simulink model "SWC_ADM"  (R2020a)
settings: Solver=FixedStepDiscrete  StartTime=0.0  StopTime=10  FixedStep=0.001  RelTol=1e-3
values from neighbouring files (symbols this model uses):
  CAL_ADM_BMSLowerThr_f32 = 0.0    [SWC_ADM_DataDictionary.sldd]
  CAL_ADM_BMSUpperThr_f32 = 0.0    [SWC_ADM_DataDictionary.sldd]
  CAL_ADM_BMSVoltRngErrCntThr_s16 = 0.0    [SWC_ADM_DataDictionary.sldd]
  CAL_ADM_BMSVoltRngErrDebThr_s16 = 0.0    [SWC_ADM_DataDictionary.sldd]
  CAL_ADM_BMSVoltRngErrRst_b = 0.0    [SWC_ADM_DataDictionary.sldd]
  CAL_ADM_DchgMode_u8 = 0.0    [SWC_ADM_DataDictionary.sldd]
  CAL_ADM_flgCrash_b = 0.0    [SWC_ADM_DataDictionary.sldd]
  CAL_ADM_flgCrashSwt_b = 0.0    [SWC_ADM_DataDictionary.sldd]
  CAL_ADM_flgDchgReq_b = 0.0    [SWC_ADM_DataDictionary.sldd]
  CAL_ADM_flgDchgReqSwt_b = 0.0    [SWC_ADM_DataDictionary.sldd]
  CAL_ADM_flgstModeReqSwt_b = 0.0    [SWC_ADM_DataDictionary.sldd]
  CAL_ADM_GlbDchgErrRst_b = 0.0    [SWC_ADM_DataDictionary.sldd]
  CAL_ADM_GlbDchgThrshTime_f32 = 0.0    [SWC_ADM_DataDictionary.sldd]
  CAL_ADM_GlbDchgThrshVolt_f32 = 0.0    [SWC_ADM_DataDictionary.sldd]
  CAL_ADM_L2Com_BMSVolt = 0.0    [SWC_ADM_DataDictionary.sldd]
  CAL_ADM_L2Com_BMSVolt_b = 0.0    [SWC_ADM_DataDictionary.sldd]
  CAL_ADM_L2Com_HiPrecVolt = 0.0    [SWC_ADM_DataDictionary.sldd]
  CAL_ADM_L2Com_HiPrecVolt_b = 0.0    [SWC_ADM_DataDictionary.sldd]
  CAL_ADM_stModeReq_u8 = 0.0    [SWC_ADM_DataDictionary.sldd]
  CAL_ADM_VoltAbsDiffThr_f32 = 0.0    [SWC_ADM_DataDictionary.sldd]
  CAL_ADM_VoltAbsDiffThrPerc_f32 = 0.0    [SWC_ADM_DataDictionary.sldd]
  CAL_ADM_VoltChgThr_f32 = 0.0    [SWC_ADM_DataDictionary.sldd]
  CAL_ADM_VoltCmpChkErrCntThr_s16 = 0.0    [SWC_ADM_DataDictionary.sldd]
  CAL_ADM_VoltCmpChkErrDebThr_s16 = 0.0    [SWC_ADM_DataDictionary.sldd]
  CAL_ADM_VoltCmpChkErrRst_b = 0.0    [SWC_ADM_DataDictionary.sldd]
  CAL_ADM_VoltCmpChkErrst_b = 0.0    [SWC_ADM_DataDictionary.sldd]
libraries: simulink x2
settings Model: DataDictionary=SWC_ADM_DataDictionary.sldd  Creator=wangzeda  LastModifiedBy=yangxinqiao
settings DataIOCC: SaveFormat=StructureWithTime
settings OptimizationCC: DefaultParameterBehavior=Inlined  DefaultUnderspecifiedDataType=single  EnhancedBackFolding=on  PassReuseOutputArgsAs=Individual arguments  ZeroExternalMemoryAtStartup=off  ZeroInternalMemoryAtStartup=off  OptimizeBlockOrder=speed  DifferentSizesBufferReuse=on  OptimizationCustomize=off  EfficientTunableParamExpr=on
settings DebuggingCC: ParameterTunabilityLossMsg=error
settings ModelReferenceCC: ModelReferenceNumInstancesAllowed=Single
settings SFSimCC: MATLABDynamicMemAlloc=off
settings RTWCC: SystemTargetFile=ert.tlc  GenCodeOnly=on  TemplateMakefile=ert_default_tmf  CustomSourceCode="#include \"set_get_data.h\""
settings CodeAppCC: ForceParamTrailComments=on  IgnoreCustomStorageClasses=off  OperatorAnnotations=on  SimulinkDataObjDesc=on  SFDataObjDesc=on  InsertBlockDesc=on
settings ERTTargetCC: TargetLangStandard=C99 (ISO)  GenerateASAP2=on  InlinedParameterPlacement=NonHierarchical  ERTCustomFileTemplate=example_file_process.tlc  EnableUserReplacementTypes=on

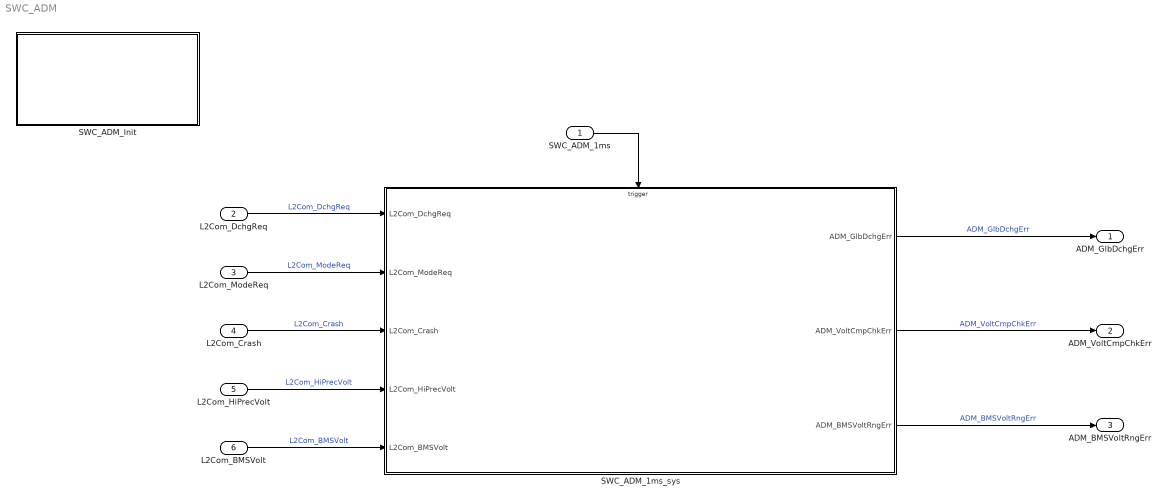
== system SWC_ADM ==
  SWC_ADM_1ms : Inport  SampleTime=0.001  OutputFunctionCall=on
  L2Com_DchgReq : Inport  Port=2  OutDataTypeStr=boolean  PortDimensions=1
  L2Com_ModeReq : Inport  Port=3  OutDataTypeStr=uint8  PortDimensions=1
  L2Com_Crash : Inport  Port=4  OutDataTypeStr=boolean  PortDimensions=1
  L2Com_HiPrecVolt : Inport  Port=5  OutDataTypeStr=single  PortDimensions=1
  L2Com_BMSVolt : Inport  Port=6  OutDataTypeStr=single  PortDimensions=1
  SWC_ADM_1ms_sys : Subsystem
  SWC_ADM_Init : Subsystem
  ADM_GlbDchgErr : Outport  OutDataTypeStr=boolean  PortDimensions=1
  ADM_VoltCmpChkErr : Outport  Port=2  OutDataTypeStr=boolean  OutputWhenDisabled=reset  InitialOutput=[0]  VectorParamsAs1DForOutWhenUnconnected=off
  ADM_BMSVoltRngErr : Outport  Port=3  OutDataTypeStr=boolean  PortDimensions=1
  wires:
  L2Com_Crash/1 -> SWC_ADM_1ms_sys/3(L2Com_Crash)  "L2Com_Crash"
  L2Com_BMSVolt/1 -> SWC_ADM_1ms_sys/5(L2Com_BMSVolt)  "L2Com_BMSVolt"
  SWC_ADM_1ms_sys/1(ADM_GlbDchgErr) -> ADM_GlbDchgErr/1  "ADM_GlbDchgErr"
  SWC_ADM_1ms/1 -> SWC_ADM_1ms_sys/Trigger
  L2Com_ModeReq/1 -> SWC_ADM_1ms_sys/2(L2Com_ModeReq)  "L2Com_ModeReq"
  L2Com_DchgReq/1 -> SWC_ADM_1ms_sys/1(L2Com_DchgReq)  "L2Com_DchgReq"
  SWC_ADM_1ms_sys/3(ADM_BMSVoltRngErr) -> ADM_BMSVoltRngErr/1  "ADM_BMSVoltRngErr"
  L2Com_HiPrecVolt/1 -> SWC_ADM_1ms_sys/4(L2Com_HiPrecVolt)  "L2Com_HiPrecVolt"
  SWC_ADM_1ms_sys/2(ADM_VoltCmpChkErr) -> ADM_VoltCmpChkErr/1  "ADM_VoltCmpChkErr"

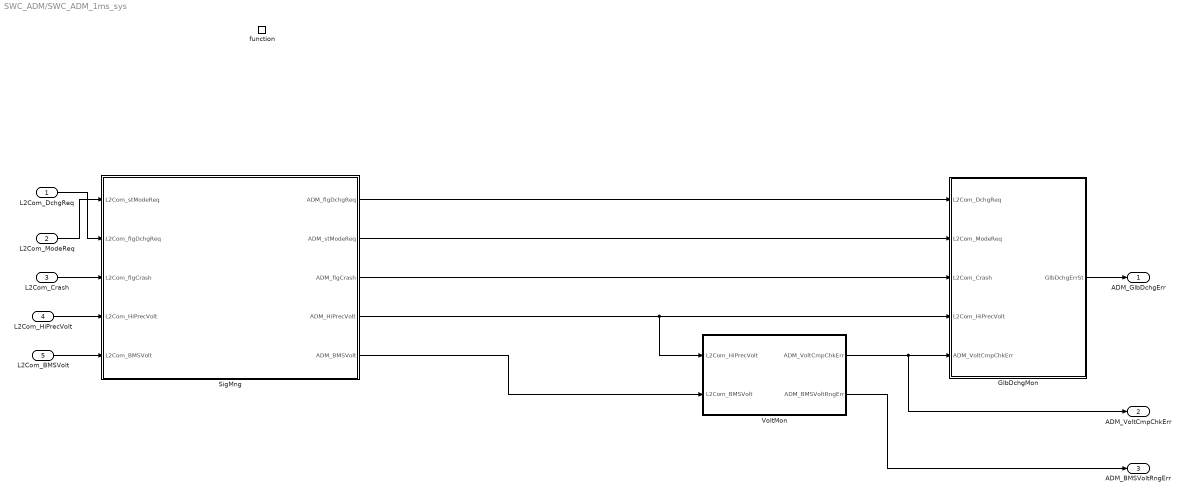
== system SWC_ADM/SWC_ADM_1ms_sys ==
  L2Com_DchgReq : Inport
  L2Com_ModeReq : Inport  Port=2
  L2Com_Crash : Inport  Port=3
  L2Com_HiPrecVolt : Inport  Port=4
  L2Com_BMSVolt : Inport  Port=5
  function : TriggerPort  TriggerType=function-call  VariantControl=(inherit)  SampleTimeType=periodic  SampleTime=-1
  GlbDchgMon : Subsystem  TreatAsAtomicUnit=on
      settings: RTWSystemCode=Nonreusable function
  SigMng : Subsystem  TreatAsAtomicUnit=on
  VoltMon : Subsystem
      settings: RTWSystemCode=Nonreusable function
  ADM_GlbDchgErr : Outport  VectorParamsAs1DForOutWhenUnconnected=off
  ADM_VoltCmpChkErr : Outport  Port=2  OutDataTypeStr=boolean  OutputWhenDisabled=reset  InitialOutput=[0]  VectorParamsAs1DForOutWhenUnconnected=off
  ADM_BMSVoltRngErr : Outport  Port=3  VectorParamsAs1DForOutWhenUnconnected=off
  wires:
  GlbDchgMon/1(GlbDchgErrSt) -> ADM_GlbDchgErr/1
  VoltMon/2(ADM_BMSVoltRngErr) -> ADM_BMSVoltRngErr/1
  VoltMon/1(ADM_VoltCmpChkErr) -> ADM_VoltCmpChkErr/1, GlbDchgMon/5(ADM_VoltCmpChkErr)
  SigMng/3(ADM_flgCrash) -> GlbDchgMon/3(L2Com_Crash)
  SigMng/2(ADM_stModeReq) -> GlbDchgMon/2(L2Com_ModeReq)
  SigMng/1(ADM_flgDchgReq) -> GlbDchgMon/1(L2Com_DchgReq)
  SigMng/4(ADM_HiPrecVolt) -> VoltMon/1(L2Com_HiPrecVolt), GlbDchgMon/4(L2Com_HiPrecVolt)
  SigMng/5(ADM_BMSVolt) -> VoltMon/2(L2Com_BMSVolt)
  L2Com_DchgReq/1 -> SigMng/2(L2Com_flgDchgReq)
  L2Com_ModeReq/1 -> SigMng/1(L2Com_stModeReq)
  L2Com_Crash/1 -> SigMng/3(L2Com_flgCrash)
  L2Com_HiPrecVolt/1 -> SigMng/4(L2Com_HiPrecVolt)
  L2Com_BMSVolt/1 -> SigMng/5(L2Com_BMSVolt)

== system SWC_ADM/SWC_ADM_Init ==
  Event Listener : EventListener  EventName=reset

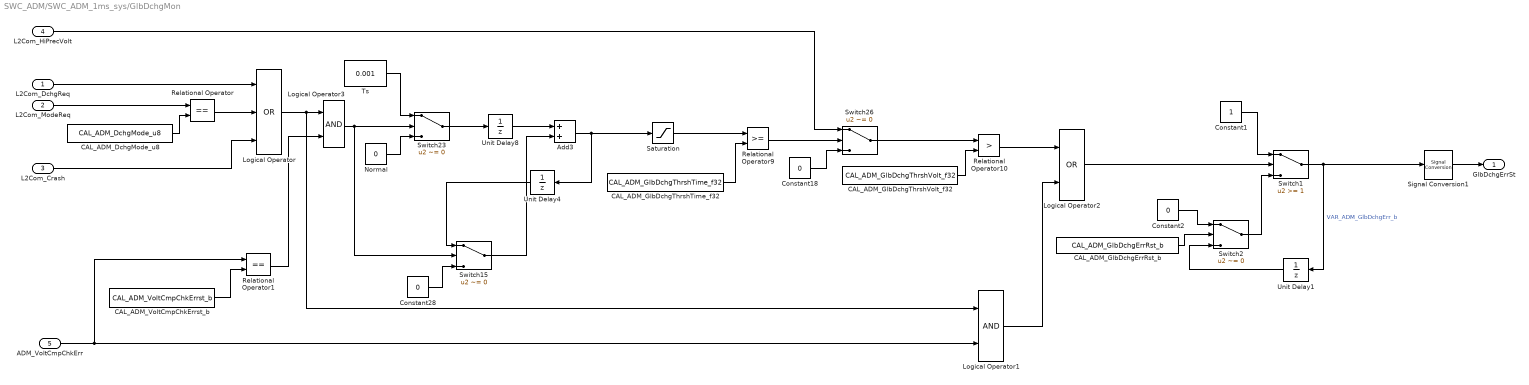
== system SWC_ADM/SWC_ADM_1ms_sys/GlbDchgMon ==
  L2Com_DchgReq : Inport
  L2Com_ModeReq : Inport  Port=2
  L2Com_Crash : Inport  Port=3
  L2Com_HiPrecVolt : Inport  Port=4
  ADM_VoltCmpChkErr : Inport  Port=5
  Add3 : Sum  AccumDataTypeStr=single
  CAL_ADM_DchgMode_u8 : Constant  Value=CAL_ADM_DchgMode_u8
  CAL_ADM_GlbDchgErrRst_b : Constant  Value=CAL_ADM_GlbDchgErrRst_b
  CAL_ADM_GlbDchgThrshTime_f32 : Constant  Value=CAL_ADM_GlbDchgThrshTime_f32
  CAL_ADM_GlbDchgThrshVolt_f32 : Constant  Value=CAL_ADM_GlbDchgThrshVolt_f32
  CAL_ADM_VoltCmpChkErrst_b : Constant  Value=CAL_ADM_VoltCmpChkErrst_b
  Constant1 : Constant  OutDataTypeStr=boolean
  Constant18 : Constant  Value=0
  Constant2 : Constant  Value=0  OutDataTypeStr=boolean
  Constant28 : Constant  Value=0
  Logical Operator : Logic  Operator=OR  Inputs=3  AllPortsSameDT=off  OutDataTypeStr=boolean
  Logical Operator1 : Logic  AllPortsSameDT=off  OutDataTypeStr=boolean
  Logical Operator2 : Logic  Operator=OR  AllPortsSameDT=off  OutDataTypeStr=boolean
  Logical Operator3 : Logic  AllPortsSameDT=off  OutDataTypeStr=boolean
  Normal : Constant  Value=0
  Relational Operator : RelationalOperator  Operator===  OutDataTypeStr=boolean  RndMeth=Simplest
  Relational Operator1 : RelationalOperator  Operator===  OutDataTypeStr=boolean  RndMeth=Simplest
  Relational Operator10 : RelationalOperator  Operator=>  OutDataTypeStr=boolean  RndMeth=Simplest
  Relational Operator9 : RelationalOperator  OutDataTypeStr=boolean  RndMeth=Simplest
  Saturation : Saturate  UpperLimit=3  LowerLimit=0
  Signal Conversion1 : SignalConversion  OverrideOpt=off
  Switch1 : Switch  Threshold=1
  Switch15 : Switch  Criteria=u2 ~= 0  OutDataTypeStr=single
  Switch2 : Switch  Criteria=u2 ~= 0
  Switch23 : Switch  Criteria=u2 ~= 0  OutDataTypeStr=single
  Switch26 : Switch  Criteria=u2 ~= 0  OutDataTypeStr=single
  Ts : Constant  Value=0.001
  Unit Delay1 : UnitDelay  SampleTime=-1  HasFrameUpgradeWarning=on
  Unit Delay4 : UnitDelay  SampleTime=-1  HasFrameUpgradeWarning=on
  Unit Delay8 : UnitDelay  SampleTime=-1  HasFrameUpgradeWarning=on
  GlbDchgErrSt : Outport  OutDataTypeStr=boolean  OutputWhenDisabled=reset  InitialOutput=[0]  VectorParamsAs1DForOutWhenUnconnected=off
  wires:
  Switch26/1 -> Relational Operator10/1
  Unit Delay4/1 -> Switch15/1
  Constant18/1 -> Switch26/3
  CAL_ADM_GlbDchgThrshVolt_f32/1 -> Relational Operator10/2
  Unit Delay8/1 -> Add3/1
  Logical Operator/1 -> Logical Operator1/1, Logical Operator3/1
  Constant28/1 -> Switch15/3
  Unit Delay1/1 -> Switch2/3
  Add3/1 -> Saturation/1, Unit Delay4/1
  Switch15/1 -> Add3/2
  Switch23/1 -> Unit Delay8/1
  Normal/1 -> Switch23/3
  Ts/1 -> Switch23/1
  Saturation/1 -> Relational Operator9/1
  CAL_ADM_GlbDchgThrshTime_f32/1 -> Relational Operator9/2
  Constant2/1 -> Switch2/1
  CAL_ADM_GlbDchgErrRst_b/1 -> Switch2/2
  L2Com_HiPrecVolt/1 -> Switch26/1
  Relational Operator10/1 -> Logical Operator2/1
  Signal Conversion1/1 -> GlbDchgErrSt/1
  Relational Operator9/1 -> Switch26/2
  L2Com_DchgReq/1 -> Logical Operator/1
  CAL_ADM_DchgMode_u8/1 -> Relational Operator/2
  L2Com_Crash/1 -> Logical Operator/3
  Relational Operator/1 -> Logical Operator/2
  L2Com_ModeReq/1 -> Relational Operator/1
  ADM_VoltCmpChkErr/1 -> Logical Operator1/2, Relational Operator1/1
  Logical Operator1/1 -> Logical Operator2/2
  Switch1/1 -> Unit Delay1/1, Signal Conversion1/1  "VAR_ADM_GlbDchgErr_b"
  CAL_ADM_VoltCmpChkErrst_b/1 -> Relational Operator1/2
  Relational Operator1/1 -> Logical Operator3/2
  Logical Operator3/1 -> Switch15/2, Switch23/2
  Logical Operator2/1 -> Switch1/2
  Constant1/1 -> Switch1/1
  Switch2/1 -> Switch1/3

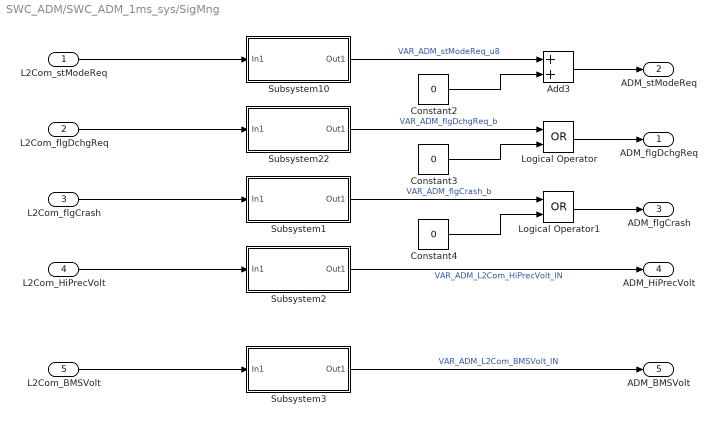
== system SWC_ADM/SWC_ADM_1ms_sys/SigMng ==
  L2Com_stModeReq : Inport
  L2Com_flgDchgReq : Inport  Port=2
  L2Com_flgCrash : Inport  Port=3
  L2Com_HiPrecVolt : Inport  Port=4
  L2Com_BMSVolt : Inport  Port=5
  Add3 : Sum
  Constant2 : Constant  Value=0  OutDataTypeStr=uint8
  Constant3 : Constant  Value=0  OutDataTypeStr=boolean
  Constant4 : Constant  Value=0  OutDataTypeStr=boolean
  Logical Operator : Logic  Operator=OR  AllPortsSameDT=off  OutDataTypeStr=boolean
  Logical Operator1 : Logic  Operator=OR  AllPortsSameDT=off  OutDataTypeStr=boolean
  Subsystem1 : Subsystem  mask{Switch_C=CAL_ADM_flgCrashSwt_b, Phy_Signal_C=CAL_ADM_flgCrash_b}
      mask prompts: Switch_C "Swich_C"
  Subsystem10 : Subsystem  mask{Switch_C=CAL_ADM_flgstModeReqSwt_b, Phy_Signal_C=CAL_ADM_stModeReq_u8}
      mask prompts: Switch_C "Swich_C"
  Subsystem2 : Subsystem  mask{Switch_C=CAL_ADM_L2Com_HiPrecVolt_b, Phy_Signal_C=CAL_ADM_L2Com_HiPrecVolt}
      mask prompts: Switch_C "Swich_C"
  Subsystem22 : Subsystem  mask{Switch_C=CAL_ADM_flgDchgReqSwt_b, Phy_Signal_C=CAL_ADM_flgDchgReq_b}
      mask prompts: Switch_C "Swich_C"
  Subsystem3 : Subsystem  mask{Switch_C=CAL_ADM_L2Com_BMSVolt_b, Phy_Signal_C=CAL_ADM_L2Com_BMSVolt}
      mask prompts: Switch_C "Swich_C"
  ADM_flgDchgReq : Outport  OutDataTypeStr=boolean  PortDimensions=1
  ADM_stModeReq : Outport  Port=2  OutDataTypeStr=uint8  PortDimensions=1
  ADM_flgCrash : Outport  Port=3  OutDataTypeStr=boolean  PortDimensions=1
  ADM_HiPrecVolt : Outport  Port=4
  ADM_BMSVolt : Outport  Port=5
  wires:
  Subsystem1/1(Out1) -> Logical Operator1/1  "VAR_ADM_flgCrash_b"
  Add3/1 -> ADM_stModeReq/1
  L2Com_flgCrash/1 -> Subsystem1/1(In1)
  Constant3/1 -> Logical Operator/2
  L2Com_flgDchgReq/1 -> Subsystem22/1(In1)
  Constant2/1 -> Add3/2
  Logical Operator/1 -> ADM_flgDchgReq/1
  Constant4/1 -> Logical Operator1/2
  Logical Operator1/1 -> ADM_flgCrash/1
  L2Com_stModeReq/1 -> Subsystem10/1(In1)
  Subsystem10/1(Out1) -> Add3/1  "VAR_ADM_stModeReq_u8"
  Subsystem22/1(Out1) -> Logical Operator/1  "VAR_ADM_flgDchgReq_b"
  L2Com_HiPrecVolt/1 -> Subsystem2/1(In1)
  Subsystem2/1(Out1) -> ADM_HiPrecVolt/1  "VAR_ADM_L2Com_HiPrecVolt_IN"
  L2Com_BMSVolt/1 -> Subsystem3/1(In1)
  Subsystem3/1(Out1) -> ADM_BMSVolt/1  "VAR_ADM_L2Com_BMSVolt_IN"

== system SWC_ADM/SWC_ADM_1ms_sys/VoltMon ==
  L2Com_HiPrecVolt : Inport
  L2Com_BMSVolt : Inport  Port=2
  BMSVoltRngMon : Subsystem
      settings: RTWSystemCode=Nonreusable function
  VoltCmpChkMon : Subsystem
      settings: RTWSystemCode=Nonreusable function
  ADM_VoltCmpChkErr : Outport  OutDataTypeStr=boolean  OutputWhenDisabled=reset  InitialOutput=[0]  VectorParamsAs1DForOutWhenUnconnected=off
  ADM_BMSVoltRngErr : Outport  Port=2  OutDataTypeStr=boolean  OutputWhenDisabled=reset  InitialOutput=[0]  VectorParamsAs1DForOutWhenUnconnected=off
  wires:
  BMSVoltRngMon/1(ADM_BMSVoltRngErr) -> ADM_BMSVoltRngErr/1
  L2Com_HiPrecVolt/1 -> VoltCmpChkMon/1(L2Com_HiPrecVolt)
  VoltCmpChkMon/1(ADM_VoltCmpChkErr) -> ADM_VoltCmpChkErr/1
  L2Com_BMSVolt/1 -> BMSVoltRngMon/1(L2Com_BMSVolt), VoltCmpChkMon/2(L2Com_BMSVolt)

== system SWC_ADM/SWC_ADM_1ms_sys/SigMng/Subsystem1 ==
  In1 : Inport
  Constant2 : Constant  Value=Switch_C  OutDataTypeStr=boolean
  Constant3 : Constant  Value=Phy_Signal_C
  Data Type Conversion : DataTypeConversion
  Switch : Switch  Criteria=u2 ~= 0
  Out1 : Outport  VectorParamsAs1DForOutWhenUnconnected=off
  wires:
  Data Type Conversion/1 -> Switch/3
  Constant3/1 -> Switch/1
  In1/1 -> Data Type Conversion/1
  Constant2/1 -> Switch/2
  Switch/1 -> Out1/1

== system SWC_ADM/SWC_ADM_1ms_sys/SigMng/Subsystem10 ==
  In1 : Inport
  Constant2 : Constant  Value=Switch_C  OutDataTypeStr=boolean
  Constant3 : Constant  Value=Phy_Signal_C
  Data Type Conversion : DataTypeConversion
  Switch : Switch  Criteria=u2 ~= 0
  Out1 : Outport  VectorParamsAs1DForOutWhenUnconnected=off
  wires:
  Switch/1 -> Out1/1
  Constant2/1 -> Switch/2
  In1/1 -> Data Type Conversion/1
  Constant3/1 -> Switch/1
  Data Type Conversion/1 -> Switch/3

== system SWC_ADM/SWC_ADM_1ms_sys/SigMng/Subsystem2 ==
  In1 : Inport
  Constant2 : Constant  Value=Switch_C  OutDataTypeStr=boolean
  Constant3 : Constant  Value=Phy_Signal_C
  Data Type Conversion : DataTypeConversion
  Switch : Switch  Criteria=u2 ~= 0
  Out1 : Outport  VectorParamsAs1DForOutWhenUnconnected=off
  wires:
  Data Type Conversion/1 -> Switch/3
  Constant3/1 -> Switch/1
  In1/1 -> Data Type Conversion/1
  Constant2/1 -> Switch/2
  Switch/1 -> Out1/1

== system SWC_ADM/SWC_ADM_1ms_sys/SigMng/Subsystem22 ==
  In1 : Inport
  Constant2 : Constant  Value=Switch_C  OutDataTypeStr=boolean
  Constant3 : Constant  Value=Phy_Signal_C
  Data Type Conversion : DataTypeConversion
  Switch : Switch  Criteria=u2 ~= 0
  Out1 : Outport  VectorParamsAs1DForOutWhenUnconnected=off
  wires:
  Switch/1 -> Out1/1
  Constant2/1 -> Switch/2
  In1/1 -> Data Type Conversion/1
  Constant3/1 -> Switch/1
  Data Type Conversion/1 -> Switch/3

== system SWC_ADM/SWC_ADM_1ms_sys/SigMng/Subsystem3 ==
  In1 : Inport
  Constant2 : Constant  Value=Switch_C  OutDataTypeStr=boolean
  Constant3 : Constant  Value=Phy_Signal_C
  Data Type Conversion : DataTypeConversion
  Switch : Switch  Criteria=u2 ~= 0
  Out1 : Outport  VectorParamsAs1DForOutWhenUnconnected=off
  wires:
  Data Type Conversion/1 -> Switch/3
  Constant3/1 -> Switch/1
  In1/1 -> Data Type Conversion/1
  Constant2/1 -> Switch/2
  Switch/1 -> Out1/1

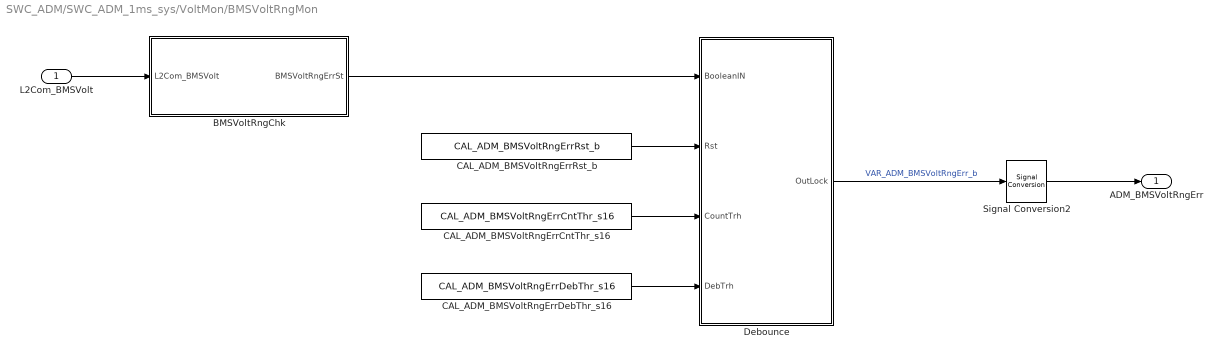
== system SWC_ADM/SWC_ADM_1ms_sys/VoltMon/BMSVoltRngMon ==
  L2Com_BMSVolt : Inport
  BMSVoltRngChk : Subsystem  TreatAsAtomicUnit=on
      settings: RTWSystemCode=Nonreusable function
  CAL_ADM_BMSVoltRngErrCntThr_s16 : Constant  Value=CAL_ADM_BMSVoltRngErrCntThr_s16  OutDataTypeStr=int16
  CAL_ADM_BMSVoltRngErrDebThr_s16 : Constant  Value=CAL_ADM_BMSVoltRngErrDebThr_s16  OutDataTypeStr=int16
  CAL_ADM_BMSVoltRngErrRst_b : Constant  Value=CAL_ADM_BMSVoltRngErrRst_b  OutDataTypeStr=boolean
  Debounce : Subsystem  TreatAsAtomicUnit=on
  Signal Conversion2 : SignalConversion  OverrideOpt=off
  ADM_BMSVoltRngErr : Outport  OutDataTypeStr=boolean  OutputWhenDisabled=reset  InitialOutput=[0]  VectorParamsAs1DForOutWhenUnconnected=off
  wires:
  L2Com_BMSVolt/1 -> BMSVoltRngChk/1(L2Com_BMSVolt)
  Signal Conversion2/1 -> ADM_BMSVoltRngErr/1
  CAL_ADM_BMSVoltRngErrRst_b/1 -> Debounce/2(Rst)
  BMSVoltRngChk/1(BMSVoltRngErrSt) -> Debounce/1(BooleanIN)
  CAL_ADM_BMSVoltRngErrDebThr_s16/1 -> Debounce/4(DebTrh)
  Debounce/1(OutLock) -> Signal Conversion2/1  "VAR_ADM_BMSVoltRngErr_b"
  CAL_ADM_BMSVoltRngErrCntThr_s16/1 -> Debounce/3(CountTrh)

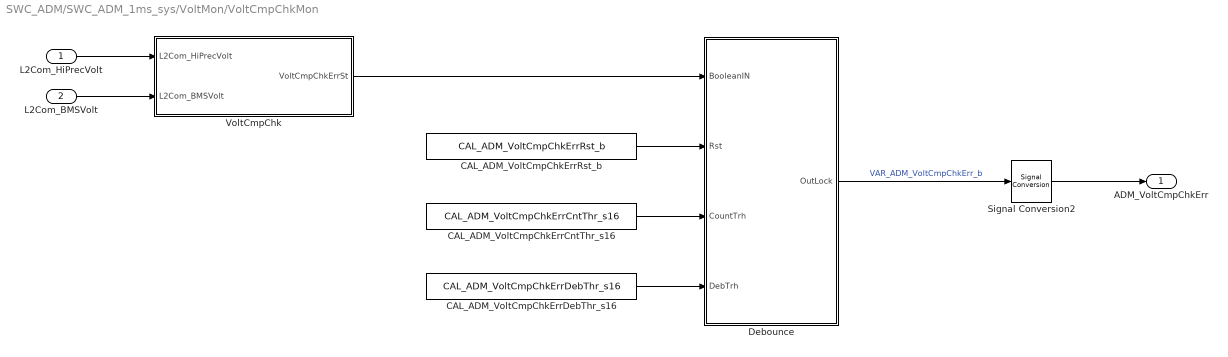
== system SWC_ADM/SWC_ADM_1ms_sys/VoltMon/VoltCmpChkMon ==
  L2Com_HiPrecVolt : Inport
  L2Com_BMSVolt : Inport  Port=2
  CAL_ADM_VoltCmpChkErrCntThr_s16 : Constant  Value=CAL_ADM_VoltCmpChkErrCntThr_s16  OutDataTypeStr=int16
  CAL_ADM_VoltCmpChkErrDebThr_s16 : Constant  Value=CAL_ADM_VoltCmpChkErrDebThr_s16  OutDataTypeStr=int16
  CAL_ADM_VoltCmpChkErrRst_b : Constant  Value=CAL_ADM_VoltCmpChkErrRst_b  OutDataTypeStr=boolean
  Debounce : Subsystem  TreatAsAtomicUnit=on
  Signal Conversion2 : SignalConversion  OverrideOpt=off
  VoltCmpChk : Subsystem  TreatAsAtomicUnit=on
      settings: RTWSystemCode=Nonreusable function
  ADM_VoltCmpChkErr : Outport  OutDataTypeStr=boolean  OutputWhenDisabled=reset  InitialOutput=[0]  VectorParamsAs1DForOutWhenUnconnected=off
  wires:
  L2Com_HiPrecVolt/1 -> VoltCmpChk/1(L2Com_HiPrecVolt)
  Signal Conversion2/1 -> ADM_VoltCmpChkErr/1
  CAL_ADM_VoltCmpChkErrRst_b/1 -> Debounce/2(Rst)
  VoltCmpChk/1(VoltCmpChkErrSt) -> Debounce/1(BooleanIN)
  CAL_ADM_VoltCmpChkErrDebThr_s16/1 -> Debounce/4(DebTrh)
  Debounce/1(OutLock) -> Signal Conversion2/1  "VAR_ADM_VoltCmpChkErr_b"
  CAL_ADM_VoltCmpChkErrCntThr_s16/1 -> Debounce/3(CountTrh)
  L2Com_BMSVolt/1 -> VoltCmpChk/2(L2Com_BMSVolt)

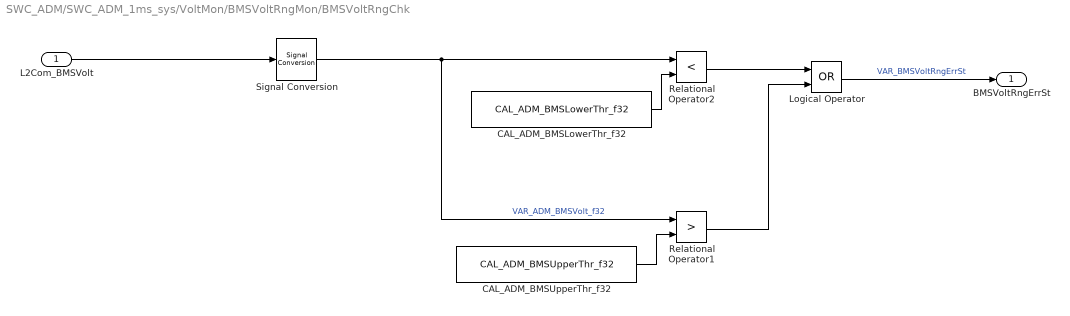
== system SWC_ADM/SWC_ADM_1ms_sys/VoltMon/BMSVoltRngMon/BMSVoltRngChk ==
  L2Com_BMSVolt : Inport
  CAL_ADM_BMSLowerThr_f32 : Constant  Value=CAL_ADM_BMSLowerThr_f32  OutDataTypeStr=single
  CAL_ADM_BMSUpperThr_f32 : Constant  Value=CAL_ADM_BMSUpperThr_f32  OutDataTypeStr=single
  Logical Operator : Logic  Operator=OR  AllPortsSameDT=off  OutDataTypeStr=boolean
  Relational Operator1 : RelationalOperator  Operator=>  OutDataTypeStr=boolean  RndMeth=Simplest
  Relational Operator2 : RelationalOperator  Operator=<  OutDataTypeStr=boolean  RndMeth=Simplest
  Signal Conversion : SignalConversion  OverrideOpt=off
  BMSVoltRngErrSt : Outport
  wires:
  Logical Operator/1 -> BMSVoltRngErrSt/1  "VAR_BMSVoltRngErrSt"
  Relational Operator1/1 -> Logical Operator/2
  Relational Operator2/1 -> Logical Operator/1
  Signal Conversion/1 -> Relational Operator1/1, Relational Operator2/1  "VAR_ADM_BMSVolt_f32"
  CAL_ADM_BMSUpperThr_f32/1 -> Relational Operator1/2
  CAL_ADM_BMSLowerThr_f32/1 -> Relational Operator2/2
  L2Com_BMSVolt/1 -> Signal Conversion/1

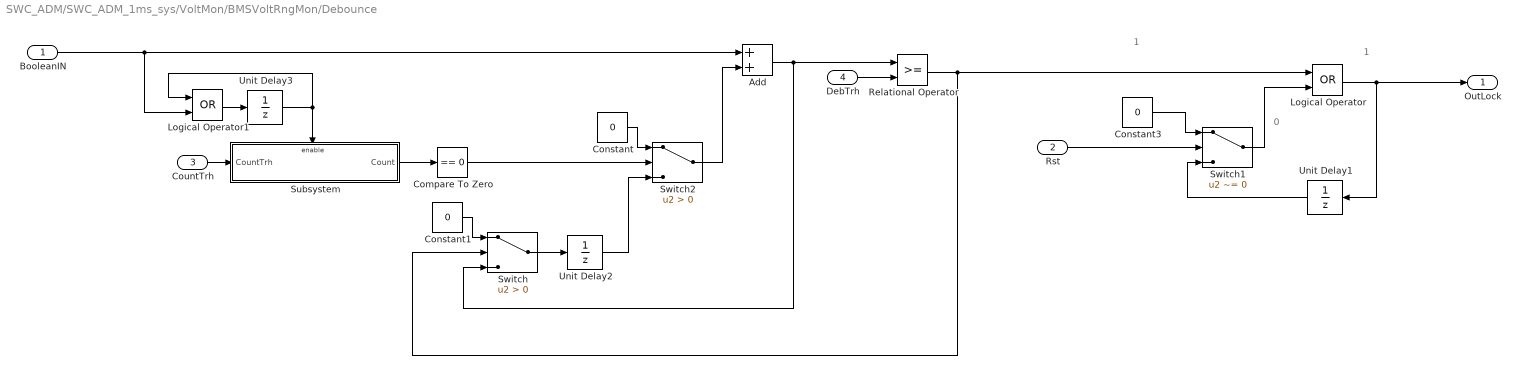
== system SWC_ADM/SWC_ADM_1ms_sys/VoltMon/BMSVoltRngMon/Debounce ==
  note: 0
  note: 1
  note: 1
  BooleanIN : Inport
  Rst : Inport  Port=2
  CountTrh : Inport  Port=3
  DebTrh : Inport  Port=4
  Add : Sum
  Compare To Zero : simulink/Logic and Bit Operations/Compare To Zero  relop===  OutDataTypeStr=boolean
  Constant : Constant  Value=0  OutDataTypeStr=int16
  Constant1 : Constant  Value=0  OutDataTypeStr=int16
  Constant3 : Constant  Value=0  OutDataTypeStr=boolean
  Logical Operator : Logic  Operator=OR  AllPortsSameDT=off  OutDataTypeStr=boolean
  Logical Operator1 : Logic  Operator=OR  AllPortsSameDT=off  OutDataTypeStr=boolean
  Relational Operator : RelationalOperator  OutDataTypeStr=boolean  RndMeth=Simplest
  Subsystem : Subsystem
  Switch : Switch  Criteria=u2 > Threshold
  Switch1 : Switch  Criteria=u2 ~= 0
  Switch2 : Switch  Criteria=u2 > Threshold
  Unit Delay1 : UnitDelay  SampleTime=-1  HasFrameUpgradeWarning=on
  Unit Delay2 : UnitDelay  SampleTime=-1  HasFrameUpgradeWarning=on
  Unit Delay3 : UnitDelay  SampleTime=-1  HasFrameUpgradeWarning=on
  OutLock : Outport  VectorParamsAs1DForOutWhenUnconnected=off
  wires:
  Constant1/1 -> Switch/1
  Add/1 -> Relational Operator/1, Switch/3
  Switch/1 -> Unit Delay2/1
  DebTrh/1 -> Relational Operator/2
  Relational Operator/1 -> Logical Operator/1, Switch/2
  BooleanIN/1 -> Add/1, Logical Operator1/2
  Unit Delay1/1 -> Switch1/3
  Switch1/1 -> Logical Operator/2
  Rst/1 -> Switch1/2
  Constant3/1 -> Switch1/1
  Logical Operator/1 -> Unit Delay1/1, OutLock/1
  Subsystem/1(Count) -> Compare To Zero/1
  Compare To Zero/1 -> Switch2/2
  Constant/1 -> Switch2/1
  Switch2/1 -> Add/2
  Unit Delay3/1 -> Logical Operator1/1, Subsystem/Enable
  Logical Operator1/1 -> Unit Delay3/1
  CountTrh/1 -> Subsystem/1(CountTrh)
  Unit Delay2/1 -> Switch2/3

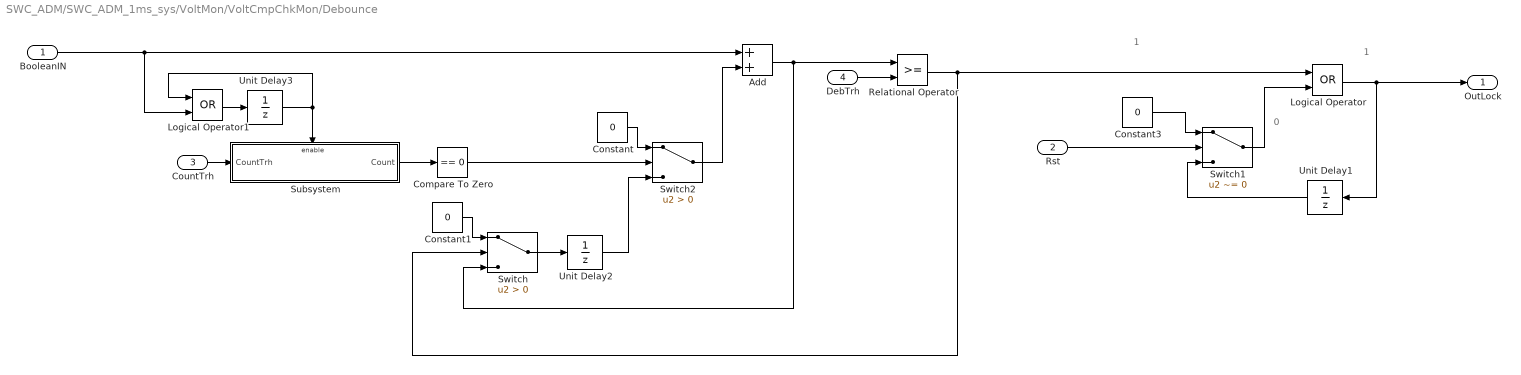
== system SWC_ADM/SWC_ADM_1ms_sys/VoltMon/VoltCmpChkMon/Debounce ==
  note: 0
  note: 1
  note: 1
  BooleanIN : Inport
  Rst : Inport  Port=2
  CountTrh : Inport  Port=3
  DebTrh : Inport  Port=4
  Add : Sum
  Compare To Zero : simulink/Logic and Bit Operations/Compare To Zero  relop===  OutDataTypeStr=boolean
  Constant : Constant  Value=0  OutDataTypeStr=int16
  Constant1 : Constant  Value=0  OutDataTypeStr=int16
  Constant3 : Constant  Value=0  OutDataTypeStr=boolean
  Logical Operator : Logic  Operator=OR  AllPortsSameDT=off  OutDataTypeStr=boolean
  Logical Operator1 : Logic  Operator=OR  AllPortsSameDT=off  OutDataTypeStr=boolean
  Relational Operator : RelationalOperator  OutDataTypeStr=boolean  RndMeth=Simplest
  Subsystem : Subsystem
  Switch : Switch  Criteria=u2 > Threshold
  Switch1 : Switch  Criteria=u2 ~= 0
  Switch2 : Switch  Criteria=u2 > Threshold
  Unit Delay1 : UnitDelay  SampleTime=-1  HasFrameUpgradeWarning=on
  Unit Delay2 : UnitDelay  SampleTime=-1  HasFrameUpgradeWarning=on
  Unit Delay3 : UnitDelay  SampleTime=-1  HasFrameUpgradeWarning=on
  OutLock : Outport  VectorParamsAs1DForOutWhenUnconnected=off
  wires:
  Constant1/1 -> Switch/1
  Add/1 -> Relational Operator/1, Switch/3
  Switch/1 -> Unit Delay2/1
  DebTrh/1 -> Relational Operator/2
  Relational Operator/1 -> Logical Operator/1, Switch/2
  BooleanIN/1 -> Add/1, Logical Operator1/2
  Unit Delay1/1 -> Switch1/3
  Switch1/1 -> Logical Operator/2
  Rst/1 -> Switch1/2
  Constant3/1 -> Switch1/1
  Logical Operator/1 -> Unit Delay1/1, OutLock/1
  Subsystem/1(Count) -> Compare To Zero/1
  Compare To Zero/1 -> Switch2/2
  Constant/1 -> Switch2/1
  Switch2/1 -> Add/2
  Unit Delay3/1 -> Logical Operator1/1, Subsystem/Enable
  Logical Operator1/1 -> Unit Delay3/1
  CountTrh/1 -> Subsystem/1(CountTrh)
  Unit Delay2/1 -> Switch2/3

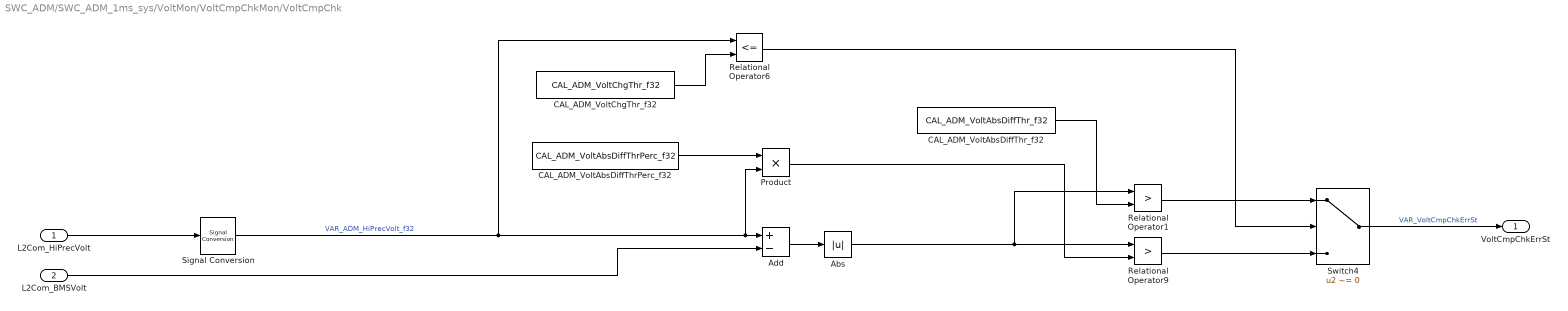
== system SWC_ADM/SWC_ADM_1ms_sys/VoltMon/VoltCmpChkMon/VoltCmpChk ==
  L2Com_HiPrecVolt : Inport
  L2Com_BMSVolt : Inport  Port=2
  Abs : Abs
  Add : Sum  Inputs=+-
  CAL_ADM_VoltAbsDiffThrPerc_f32 : Constant  Value=CAL_ADM_VoltAbsDiffThrPerc_f32  OutDataTypeStr=single
  CAL_ADM_VoltAbsDiffThr_f32 : Constant  Value=CAL_ADM_VoltAbsDiffThr_f32  OutDataTypeStr=single
  CAL_ADM_VoltChgThr_f32 : Constant  Value=CAL_ADM_VoltChgThr_f32  OutDataTypeStr=single
  Product : Product
  Relational Operator1 : RelationalOperator  Operator=>  OutDataTypeStr=boolean  RndMeth=Simplest
  Relational Operator6 : RelationalOperator  Operator=<=  OutDataTypeStr=boolean  RndMeth=Simplest
  Relational Operator9 : RelationalOperator  Operator=>  OutDataTypeStr=boolean  RndMeth=Simplest
  Signal Conversion : SignalConversion  OverrideOpt=off
  Switch4 : Switch  Criteria=u2 ~= 0
  VoltCmpChkErrSt : Outport
  wires:
  Switch4/1 -> VoltCmpChkErrSt/1  "VAR_VoltCmpChkErrSt"
  L2Com_HiPrecVolt/1 -> Signal Conversion/1
  Signal Conversion/1 -> Relational Operator6/1, Product/2, Add/1  "VAR_ADM_HiPrecVolt_f32"
  Abs/1 -> Relational Operator9/1, Relational Operator1/1
  Add/1 -> Abs/1
  CAL_ADM_VoltChgThr_f32/1 -> Relational Operator6/2
  Product/1 -> Relational Operator9/2
  CAL_ADM_VoltAbsDiffThr_f32/1 -> Relational Operator1/2
  Relational Operator9/1 -> Switch4/3
  CAL_ADM_VoltAbsDiffThrPerc_f32/1 -> Product/1
  Relational Operator1/1 -> Switch4/1
  L2Com_BMSVolt/1 -> Add/2
  Relational Operator6/1 -> Switch4/2

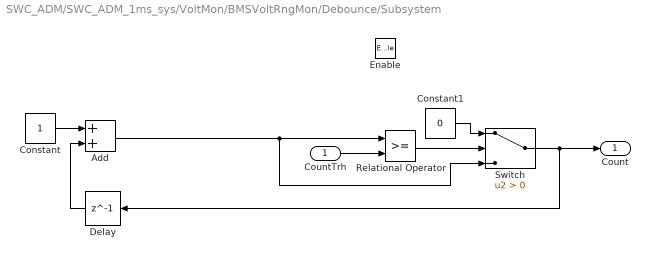
== system SWC_ADM/SWC_ADM_1ms_sys/VoltMon/BMSVoltRngMon/Debounce/Subsystem ==
  CountTrh : Inport
  Enable : EnablePort
  Add : Sum
  Constant : Constant  OutDataTypeStr=int16
  Constant1 : Constant  Value=0  OutDataTypeStr=int16
  Delay : Delay  DelayLength=1
  Relational Operator : RelationalOperator  OutDataTypeStr=boolean  RndMeth=Simplest
  Switch : Switch  Criteria=u2 > Threshold
  Count : Outport
  wires:
  Switch/1 -> Delay/1, Count/1
  Constant/1 -> Add/1
  Relational Operator/1 -> Switch/2
  Add/1 -> Relational Operator/1, Switch/3
  Constant1/1 -> Switch/1
  CountTrh/1 -> Relational Operator/2
  Delay/1 -> Add/2

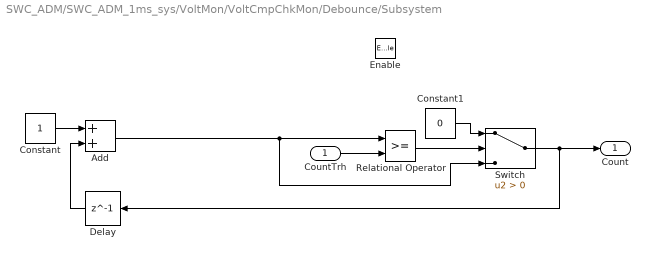
== system SWC_ADM/SWC_ADM_1ms_sys/VoltMon/VoltCmpChkMon/Debounce/Subsystem ==
  CountTrh : Inport
  Enable : EnablePort
  Add : Sum
  Constant : Constant  OutDataTypeStr=int16
  Constant1 : Constant  Value=0  OutDataTypeStr=int16
  Delay : Delay  DelayLength=1
  Relational Operator : RelationalOperator  OutDataTypeStr=boolean  RndMeth=Simplest
  Switch : Switch  Criteria=u2 > Threshold
  Count : Outport
  wires:
  Switch/1 -> Delay/1, Count/1
  Constant/1 -> Add/1
  Relational Operator/1 -> Switch/2
  Add/1 -> Relational Operator/1, Switch/3
  Constant1/1 -> Switch/1
  CountTrh/1 -> Relational Operator/2
  Delay/1 -> Add/2
